simulink model "math_vect_test"  (Simulink 7.2)
settings: Solver=VariableStepDiscrete  StartTime=0.0  StopTime=10.0  RelTol=1e-3
undefined symbols (not defined in the file or in its folder): magnitude
settings Model: Creator=arnaud  LastModifiedBy=arnaud
settings DataIOCC: SaveFormat=Structure

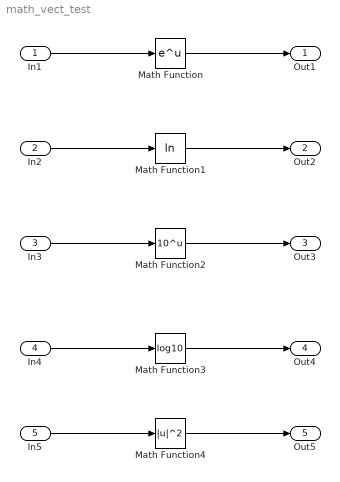
== system math_vect_test ==
  In1 : Inport  PortDimensions=3  OutDataType=sfix(16)  OutScaling=2^0
  In2 : Inport  Port=2  PortDimensions=3  OutDataType=sfix(16)  OutScaling=2^0
  In3 : Inport  Port=3  PortDimensions=3  OutDataType=sfix(16)  OutScaling=2^0
  In4 : Inport  Port=4  PortDimensions=3  OutDataType=sfix(16)  OutScaling=2^0
  In5 : Inport  Port=5  PortDimensions=3  OutDataType=sfix(16)  OutScaling=2^0
  Math Function : Math  OutDataType=sfix(16)  OutScaling=2^0  SaturateOnIntegerOverflow=on
  Math Function1 : Math  Operator=log  OutDataType=sfix(16)  OutScaling=2^0  SaturateOnIntegerOverflow=on
  Math Function2 : Math  Operator=10^u  OutDataType=sfix(16)  OutScaling=2^0  SaturateOnIntegerOverflow=on
  Math Function3 : Math  Operator=log10  OutDataType=sfix(16)  OutScaling=2^0  SaturateOnIntegerOverflow=on
  Math Function4 : Math  Operator=magnitude^2  OutDataType=sfix(16)  OutScaling=2^0  SaturateOnIntegerOverflow=on
  Out1 : Outport  OutDataType=sfix(16)  OutScaling=2^0
  Out2 : Outport  Port=2  OutDataType=sfix(16)  OutScaling=2^0
  Out3 : Outport  Port=3  OutDataType=sfix(16)  OutScaling=2^0
  Out4 : Outport  Port=4  OutDataType=sfix(16)  OutScaling=2^0
  Out5 : Outport  Port=5  OutDataType=sfix(16)  OutScaling=2^0
  wires:
  In1/1 -> Math Function/1
  Math Function/1 -> Out1/1
  In2/1 -> Math Function1/1
  Math Function1/1 -> Out2/1
  In3/1 -> Math Function2/1
  Math Function2/1 -> Out3/1
  In4/1 -> Math Function3/1
  Math Function3/1 -> Out4/1
  In5/1 -> Math Function4/1
  Math Function4/1 -> Out5/1
